simulink model "modele"  (R2023a)
settings: Solver=VariableStepAuto  StartTime=0.0  StopTime=10.0  RelTol=1e-3
settings Model: Creator=gwr2526  LastModifiedBy=gwr2526

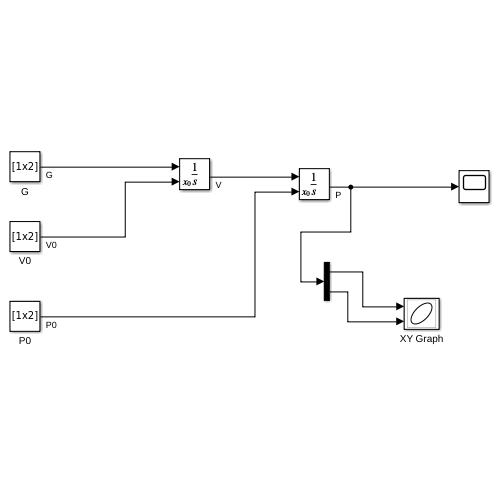
[thumbnail: Simulink's stored preview of the top-level diagram]
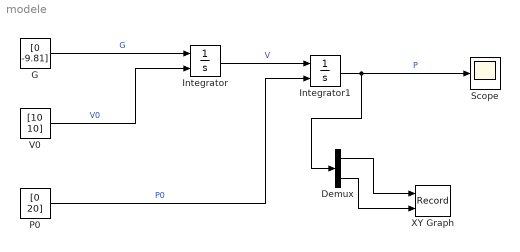
== system modele ==
  Demux : Demux  Outputs=2
  G : Constant  Value=[0 -9.81]
  Integrator : Integrator  InitialConditionSource=external
  Integrator1 : Integrator  InitialConditionSource=external
  P0 : Constant  Value=[0 20]
  Scope : Scope
  V0 : Constant  Value=[10 10]
  XY Graph : Record  FileSettingsInternal="{\"entries\":[{\"content\":{\"excelSettings\":{\"content\":{},\"type\":\"Streamout.ExcelSettings\"}},\"type\":\"Streamout.FileSettingStorage\",\"uuid\":\"ad8be83c-ecfa-4cd5-9f08-6d7b27ce661a\"}],\"packageUris\":[\"http://schema.mathworks.com/mf0/streamout_blocks/R2020a\"],\"version\":\"1.0\"}"  Layout=[1 1]  SignalsInternal="{\"entries\":[{\"content\":{\"signals\":[{\"content\":{\"blockPath\":[\"untitled/XY Graph\"],\"dimensions\":[1],\"domain\":\"untitled/XY Graph\",\"lineColor\":\"#a2142f\",\"plots\":[1],\"port\":1,\"sid\":[\"\"],\"signalID\":57,\"signalName\":\"Demux:1\"},\"type\":\"RecordBlkView.Signal\",\"uuid\":\"f2198378-3ccd-4a83-ae8a-5d885ef90d51\"},{\"content\":{\"blockPath\":[\"untitled/XY Graph\"],\"dimensions\":[1],\"domain\":\"untitled/XY Graph\",\"lineColor\":\"#139fff\",\"plots\":[1],\"port\":2,\"sid\":[\"\"],\"signalID\":61,\"signalName\":\"Demux:2\"},\"type\":\"RecordBlkView.Signal\",\"uuid\":\"592163be-1d5f-47e3-a097-792ce8ab1934\"}]},\"type\":\"RecordBlkView.InputSignals\",\"uuid\":\"14f0fefe-63d3-43b3-a6e2-3e24463827e2\"}],\"packageUris\":[\"http://schema.mathworks.com/mf0/streamout_blocks/R2020a\"],\"version\":\"1.0\"}"  VisualizationBindings="{\"xyplotplugin\":{\"info\":[{\"series\":[{\"bindingParametersList\":[{\"parameter\":\"X-Axis\",\"signalID\":57,\"signalName\":\"Demux:1\"},{\"parameter\":\"Y-Axis\",\"signalID\":61,\"signalName\":\"Demux:2\"}],\"seriesID\":62512}],\"subplotID\":1}]}}"  CompatibilityTag=XY
  wires:
  V0/1 -> Integrator/2  "V0"
  G/1 -> Integrator/1  "G"
  Integrator/1 -> Integrator1/1  "V"
  P0/1 -> Integrator1/2  "P0"
  Integrator1/1 -> Demux/1, Scope/1  "P"
  Demux/2 -> XY Graph/2
  Demux/1 -> XY Graph/1
